simulink model "process_block"  (Simulink 7.9)
settings: Solver=FixedStepDiscrete  StartTime=0.0  StopTime=1000  FixedStep=0.05  RelTol=1e-3
values from neighbouring files (symbols this model uses):
  h = 0.05    [magic_model.m]    (also in synthesize_model.m = 0.0298)
settings Model: Creator=martinka  LastModifiedBy=dat14rsa

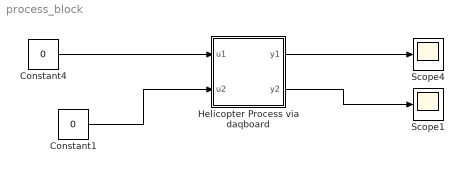
== system process_block ==
  Constant1 : Constant  Value=0  SampleTime=-1
  Constant4 : Constant  Value=0  SampleTime=-1
  Helicopter Process via daqboard : Subsystem
  Scope1 : Scope
      settings: YMin=-4  YMax=3  SaveName=ScopeData2
  Scope4 : Scope
      settings: YMin=-3.56775  YMax=-3.566
  wires:
  Helicopter Process via daqboard/1(y1) -> Scope4/1
  Helicopter Process via daqboard/2(y2) -> Scope1/1
  Constant4/1 -> Helicopter Process via daqboard/1(u1)
  Constant1/1 -> Helicopter Process via daqboard/2(u2)

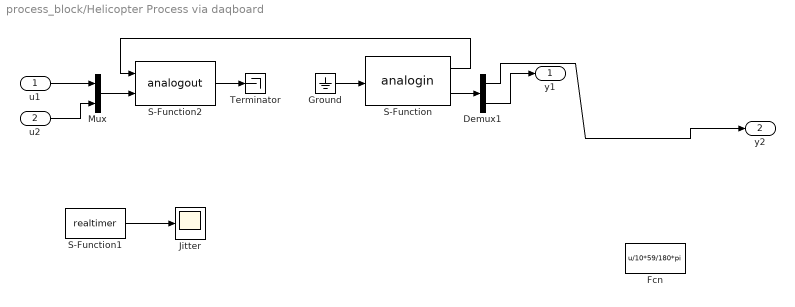
== system process_block/Helicopter Process via daqboard ==
  u1 : Inport
  u2 : Inport  Port=2
  Demux1 : Demux  Outputs=2
  Fcn : Fcn  Expr=u/10*59/180*pi
  Ground : Ground
  Jitter : Scope
  Mux : Mux  Inputs=2
  S-Function : S-Function  FunctionName=analogin  Parameters=h [0 1]  EnableBusSupport=off
  S-Function1 : S-Function  FunctionName=realtimer  Parameters=h  EnableBusSupport=off
  S-Function2 : S-Function  FunctionName=analogout  Parameters=h [0 1]  EnableBusSupport=off
  Terminator : Terminator
  y1 : Outport  InitialOutput=0
  y2 : Outport  Port=2  InitialOutput=0
  wires:
  S-Function/1 -> S-Function2/1
  S-Function2/1 -> Terminator/1
  Ground/1 -> S-Function/1
  u1/1 -> Mux/1
  u2/1 -> Mux/2
  S-Function/2 -> Demux1/1
  Demux1/2 -> y1/1
  Mux/1 -> S-Function2/2
  S-Function1/1 -> Jitter/1
  Demux1/1 -> y2/1
